simulink library "WrightSolverLib"  (R2014b)
settings: Solver=ode45  SolverMode=SingleTasking  StartTime=0.0  StopTime=10.0  RelTol=1e-3
undefined symbols (not defined in the file): BooleanThreshold, FloatingVoltage, FspSamplingPeriod, InfiniteResistance, NoCurrentOverride, WrightSolverSamplingPeriod
libraries: WrightSolverLib x34, simulink x5
settings Model: Creator=SWright2  LastModifiedBy=sj3-wright

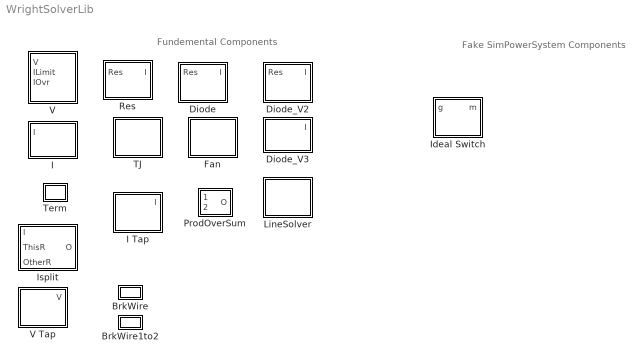
== system WrightSolverLib ==
  note: Fundemental Components
  note: Fake SimPowerSystem Components
  BrkWire : Subsystem
  BrkWire1to2 : Subsystem
  Diode : Subsystem
  Diode_V2 : Subsystem
  Diode_V3 : Subsystem
  Fan : Subsystem  RTWFcnName=TJunction  RTWFileName=TJunction
      settings: RTWFcnNameOpts=User specified  RTWFileNameOpts=User specified
  I : Subsystem
  I Tap : Subsystem
  Ideal Switch : Subsystem  mask{OnResistance=1}
  Isplit : Subsystem  RTWFcnName=Isplit  RTWFileName=Isplit
      settings: RTWFcnNameOpts=User specified  RTWFileNameOpts=User specified
  LineSolver : Subsystem
  ProdOverSum : Subsystem  RTWFcnName=ProdOverSum  RTWFileName=ProdOverSum
      settings: RTWFcnNameOpts=User specified  RTWFileNameOpts=User specified
  Res : Subsystem
  TJ : Subsystem  RTWFcnName=TJunction  RTWFileName=TJunction
      settings: RTWFcnNameOpts=User specified  RTWFileNameOpts=User specified
  Term : Subsystem
  V : Subsystem
  V Tap : Subsystem

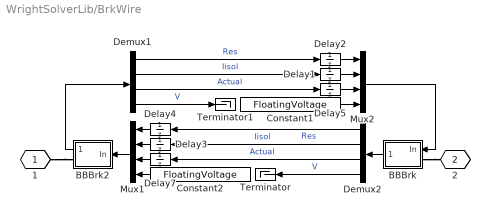
== system WrightSolverLib/BrkWire ==
  BBBrk : Subsystem
  BBBrk2 : Subsystem
  Constant1 : Constant  Value=FloatingVoltage
  Constant2 : Constant  Value=FloatingVoltage
  Delay{1,3,5,7} (4 alike) : UnitDelay  SampleTime=WrightSolverSamplingPeriod
  Delay2 : UnitDelay  InitialCondition=InfiniteResistance  SampleTime=WrightSolverSamplingPeriod
  Delay4 : UnitDelay  InitialCondition=InfiniteResistance  SampleTime=WrightSolverSamplingPeriod
  Demux1 : Demux
  Demux2 : Demux
  Mux1 : Mux
  Mux2 : Mux
  Terminator : Terminator
  Terminator1 : Terminator
  1 : PMIOPort  Tag=PMCPort  Port=1  Side=Left
  2 : PMIOPort  Tag=PMCPort  Port=2  Side=Right
  wires:
  BBBrk/1(Out) -> Demux2/1
  Demux2/3 -> Delay7/1  "Actual"
  Demux2/2 -> Delay3/1  "Iisol"
  Demux2/1 -> Delay4/1  "Res"
  Demux2/4 -> Terminator/1  "V"
  Mux1/1 -> BBBrk2/1(In)
  BBBrk2/1(Out) -> Demux1/1
  Mux2/1 -> BBBrk/1(In)
  Constant2/1 -> Mux1/4
  Delay4/1 -> Mux1/1
  Delay3/1 -> Mux1/2
  Delay7/1 -> Mux1/3
  Delay2/1 -> Mux2/1
  Delay1/1 -> Mux2/2
  Delay5/1 -> Mux2/3
  Constant1/1 -> Mux2/4
  Demux1/1 -> Delay2/1  "Res"
  Demux1/2 -> Delay1/1  "Iisol"
  Demux1/3 -> Delay5/1  "Actual"
  Demux1/4 -> Terminator1/1  "V"
  connections:
  BBBrk/LConn1 -- 2/RConn1
  1/RConn1 -- BBBrk2/RConn1

== system WrightSolverLib/BrkWire1to2 ==
  BBBrk : Subsystem
  BBBrk2 : Subsystem
  Delay : UnitDelay  InitialCondition=[InfiniteResistance 0 0 FloatingVoltage]  SampleTime=FspSamplingPeriod
  1 : PMIOPort  Tag=PMCPort  Port=1  Side=Left
  2 : PMIOPort  Tag=PMCPort  Port=2  Side=Right
  wires:
  BBBrk/1(Out) -> BBBrk2/1(In)
  BBBrk2/1(Out) -> Delay/1
  Delay/1 -> BBBrk/1(In)
  connections:
  1/RConn1 -- BBBrk2/RConn1
  BBBrk/LConn1 -- 2/RConn1

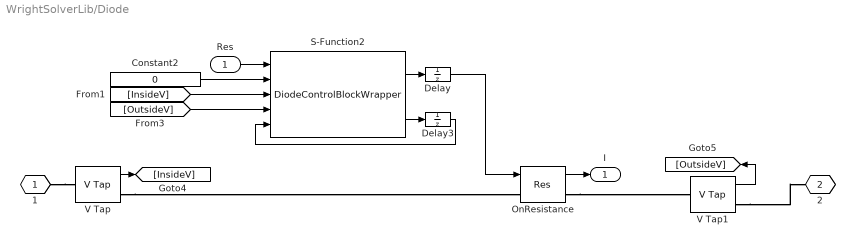
== system WrightSolverLib/Diode ==
  Res : Inport
  Constant2 : Constant  Value=0
  Delay : UnitDelay  InitialCondition=InfiniteResistance  SampleTime=-1
  Delay3 : UnitDelay  SampleTime=-1
  OnResistance : WrightSolverLib/Res
  S-Function2 : S-Function  FunctionName=DiodeControlBlockWrapper  EnableBusSupport=off
  V Tap : WrightSolverLib/V Tap
  V Tap1 : WrightSolverLib/V Tap
  1 : PMIOPort  Tag=PMCPort  Port=1  Side=Left
  2 : PMIOPort  Tag=PMCPort  Port=2  Side=Right
  I : Outport
  wires:
  V Tap1/1 -> [OutsideV]
  OnResistance/1 -> I/1
  V Tap/1 -> [InsideV]
  Constant2/1 -> S-Function2/2
  [InsideV] -> S-Function2/3
  S-Function2/1 -> Delay/1
  Res/1 -> S-Function2/1
  Delay/1 -> OnResistance/1
  S-Function2/2 -> Delay3/1
  Delay3/1 -> S-Function2/5
  [OutsideV] -> S-Function2/4
  connections:
  V Tap/RConn1 -- OnResistance/LConn1
  OnResistance/RConn1 -- V Tap1/LConn1
  1/RConn1 -- V Tap/LConn1
  V Tap1/RConn1 -- 2/RConn1

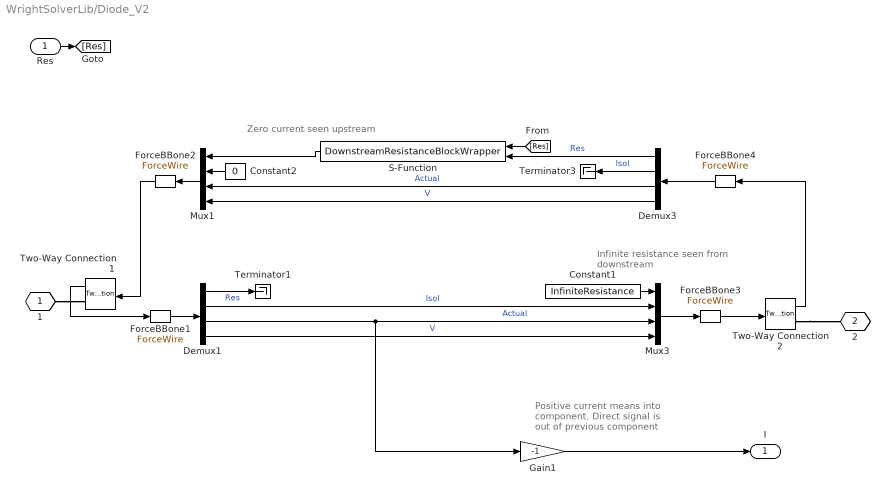
== system WrightSolverLib/Diode_V2 ==
  note: Positive current means
      | into component.
      | Direct signal is out
      | of previous
      | component
  note: Infinite
      | resistance
      | seen from
      | downstream
  note: Zero current
      | seen
      | upstream
  Res : Inport
  Constant1 : Constant  Value=InfiniteResistance
  Constant2 : Constant  Value=0
  Demux1 : Demux
  Demux3 : Demux
  ForceBBone{1..4} (4 alike) : WrightSolverLib/ForceWire
  Gain1 : Gain  Gain=-1
  Mux1 : Mux
  Mux3 : Mux
  S-Function : S-Function  FunctionName=DownstreamResistanceBlockWrapper  EnableBusSupport=off
  Terminator1 : Terminator
  Terminator3 : Terminator
  Two-Way Connection1 : TwoWayConnection
  Two-Way Connection2 : TwoWayConnection
  1 : PMIOPort  Tag=PMCPort  Port=1  Side=Left
  2 : PMIOPort  Tag=PMCPort  Port=2  Side=Right
  I : Outport
  wires:
  Gain1/1 -> I/1
  Demux3/3 -> Mux1/3  "Actual"
  Constant1/1 -> Mux3/1
  Res/1 -> [Res]
  Mux3/1 -> ForceBBone3/1
  Demux3/1 -> S-Function/2  "Res"
  Mux1/1 -> ForceBBone2/1
  S-Function/1 -> Mux1/1
  Two-Way Connection1/1 -> ForceBBone1/1
  Demux1/1 -> Terminator1/1  "Res"
  Demux3/2 -> Terminator3/1  "Isol"
  Demux1/2 -> Mux3/2  "Isol"
  Demux1/3 -> Gain1/1, Mux3/3  "Actual"
  ForceBBone2/1 -> Two-Way Connection1/1
  ForceBBone1/1 -> Demux1/1
  Constant2/1 -> Mux1/2
  Demux3/4 -> Mux1/4  "V"
  Demux1/4 -> Mux3/4  "V"
  Two-Way Connection2/1 -> ForceBBone4/1
  ForceBBone3/1 -> Two-Way Connection2/1
  ForceBBone4/1 -> Demux3/1
  [Res] -> S-Function/1
  connections:
  1/RConn1 -- Two-Way Connection1/RConn1
  Two-Way Connection2/RConn1 -- 2/RConn1

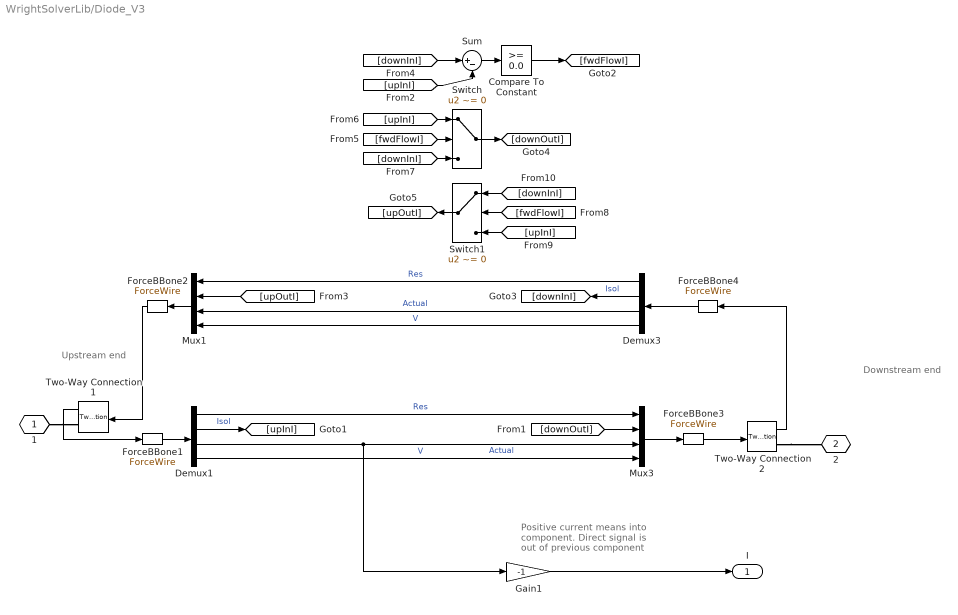
== system WrightSolverLib/Diode_V3 ==
  note: Positive current means
      | into component.
      | Direct signal is out
      | of previous
      | component
  note: Downstream
      | end
  note: Upstream
      | end
  Compare To Constant : simulink/Logic and Bit Operations/Compare To Constant  relop=>=  const=0.0  OutDataTypeStr=boolean
  Demux1 : Demux
  Demux3 : Demux
  ForceBBone{1..4} (4 alike) : WrightSolverLib/ForceWire
  Gain1 : Gain  Gain=-1
  Mux1 : Mux
  Mux3 : Mux
  Sum : Sum  Inputs=|+-
  Switch : Switch  Criteria=u2 ~= 0
  Switch1 : Switch  Criteria=u2 ~= 0
  Two-Way Connection1 : TwoWayConnection
  Two-Way Connection2 : TwoWayConnection
  1 : PMIOPort  Tag=PMCPort  Port=1  Side=Left
  2 : PMIOPort  Tag=PMCPort  Port=2  Side=Right
  I : Outport
  wires:
  Compare To Constant/1 -> [fwdFlowI]
  Sum/1 -> Compare To Constant/1
  [upInI] -> Sum/2
  [downInI] -> Sum/1
  ForceBBone4/1 -> Demux3/1
  ForceBBone3/1 -> Two-Way Connection2/1
  Two-Way Connection2/1 -> ForceBBone4/1
  Demux1/4 -> Mux3/4  "V"
  Demux3/4 -> Mux1/4  "V"
  [upOutI] -> Mux1/2
  ForceBBone1/1 -> Demux1/1
  ForceBBone2/1 -> Two-Way Connection1/1
  Demux1/3 -> Mux3/3, Gain1/1  "Actual"
  Demux3/2 -> [downInI]  "Isol"
  Demux1/1 -> Mux3/1  "Res"
  Two-Way Connection1/1 -> ForceBBone1/1
  Mux1/1 -> ForceBBone2/1
  Demux3/1 -> Mux1/1  "Res"
  Mux3/1 -> ForceBBone3/1
  Demux3/3 -> Mux1/3  "Actual"
  Gain1/1 -> I/1
  Demux1/2 -> [upInI]  "Isol"
  [downOutI] -> Mux3/2
  [fwdFlowI] -> Switch/2
  Switch/1 -> [downOutI]
  [upInI] -> Switch/1
  [downInI] -> Switch/3
  [fwdFlowI] -> Switch1/2
  Switch1/1 -> [upOutI]
  [downInI] -> Switch1/1
  [upInI] -> Switch1/3
  connections:
  Two-Way Connection2/RConn1 -- 2/RConn1
  1/RConn1 -- Two-Way Connection1/RConn1

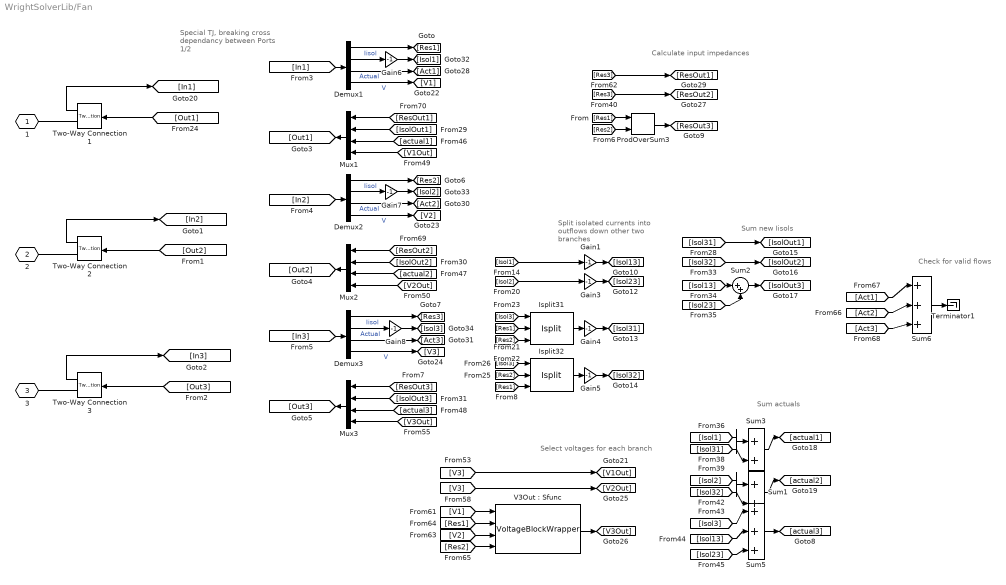
== system WrightSolverLib/Fan ==
  note: Check for valid flows
  note: Select voltages for each branch
  note: Calculate input impedances
  note: Split isolated currents
      | into outflows down other two
      | branches
  note: Sum new Iisols
  note: Sum actuals
  note: Special TJ, breaking
      | cross dependancy
      | between Ports 1/2
  Demux1 : Demux
  Demux2 : Demux
  Demux3 : Demux
  Gain{1,3..8} (7 alike) : Gain  Gain=-1
  Isplit31 : WrightSolverLib/Isplit
  Isplit32 : WrightSolverLib/Isplit
  Mux1 : Mux
  Mux2 : Mux
  Mux3 : Mux
  ProdOverSum3 : WrightSolverLib/ProdOverSum
  Sum1 : Sum  Inputs=|++
  Sum2 : Sum  Inputs=|++
  Sum3 : Sum  Inputs=|++
  Sum5 : Sum  Inputs=|+++
  Sum6 : Sum  Inputs=|+++
  Terminator1 : Terminator
  Two-Way Connection1 : TwoWayConnection
  Two-Way Connection2 : TwoWayConnection
  Two-Way Connection3 : TwoWayConnection
  "V3Out : Sfunc" : S-Function  FunctionName=VoltageBlockWrapper  EnableBusSupport=off
  1 : PMIOPort  Tag=PMCPort  Port=1  Side=Left
  2 : PMIOPort  Tag=PMCPort  Port=2  Side=Left
  3 : PMIOPort  Tag=PMCPort  Port=3  Side=Right
  wires:
  Sum6/1 -> Terminator1/1
  [Act3] -> Sum6/3
  [Act2] -> Sum6/2
  [Act1] -> Sum6/1
  Sum5/1 -> [actual3]
  Sum1/1 -> [actual2]
  Sum3/1 -> [actual1]
  "V3Out : Sfunc"/1 -> [V3Out]
  [Res2] -> "V3Out : Sfunc"/4
  [Res1] -> "V3Out : Sfunc"/2
  [V2] -> "V3Out : Sfunc"/3
  [V1] -> "V3Out : Sfunc"/1
  [V3] -> [V2Out]
  [V3] -> [V1Out]
  [V3Out] -> Mux3/4
  [V2Out] -> Mux2/4
  [V1Out] -> Mux1/4
  Mux1/1 -> [Out1]
  Mux2/1 -> [Out2]
  Mux3/1 -> [Out3]
  Demux1/1 -> [Res1]
  [Res1] -> ProdOverSum3/1
  Demux2/1 -> [Res2]
  Demux3/1 -> [Res3]
  [Res2] -> ProdOverSum3/2
  [ResOut3] -> Mux3/1
  ProdOverSum3/1 -> [ResOut3]
  [Res3] -> [ResOut2]
  [Res3] -> [ResOut1]
  [ResOut2] -> Mux2/1
  [ResOut1] -> Mux1/1
  Demux1/2 -> Gain6/1  "Iisol"
  Demux2/2 -> Gain7/1  "Iisol"
  Demux3/2 -> Gain8/1  "Iisol"
  [Isol1] -> Gain1/1
  [Isol3] -> Isplit31/1
  [Res1] -> Isplit31/2
  [Res2] -> Isplit31/3
  [Isol3] -> Isplit32/1
  [Res2] -> Isplit32/2
  [Res1] -> Isplit32/3
  [Isol31] -> [IsolOut1]
  [IsolOut1] -> Mux1/2
  [IsolOut2] -> Mux2/2
  [IsolOut3] -> Mux3/2
  [Isol32] -> [IsolOut2]
  [Isol13] -> Sum2/1
  Sum2/1 -> [IsolOut3]
  [Isol23] -> Sum2/2
  [Isol1] -> Sum3/1
  [Isol31] -> Sum3/2
  [Isol2] -> Sum1/1
  [Isol32] -> Sum1/2
  [Isol3] -> Sum5/1
  [Isol13] -> Sum5/2
  [Isol23] -> Sum5/3
  [actual1] -> Mux1/3
  [actual2] -> Mux2/3
  [actual3] -> Mux3/3
  Gain1/1 -> [Isol13]
  Gain3/1 -> [Isol23]
  Isplit31/1 -> Gain4/1
  Gain4/1 -> [Isol31]
  Isplit32/1 -> Gain5/1
  Gain5/1 -> [Isol32]
  Demux1/3 -> [Act1]  "Actual"
  Demux1/4 -> [V1]  "V"
  Demux2/3 -> [Act2]  "Actual"
  Demux2/4 -> [V2]  "V"
  Demux3/3 -> [Act3]  "Actual"
  Demux3/4 -> [V3]  "V"
  Gain6/1 -> [Isol1]
  Gain7/1 -> [Isol2]
  Gain8/1 -> [Isol3]
  [In1] -> Demux1/1
  [In2] -> Demux2/1
  [In3] -> Demux3/1
  [Out1] -> Two-Way Connection1/1
  [Out2] -> Two-Way Connection2/1
  [Out3] -> Two-Way Connection3/1
  Two-Way Connection1/1 -> [In1]
  Two-Way Connection2/1 -> [In2]
  Two-Way Connection3/1 -> [In3]
  [Isol2] -> Gain3/1
  connections:
  1/RConn1 -- Two-Way Connection1/RConn1
  2/RConn1 -- Two-Way Connection2/RConn1
  3/RConn1 -- Two-Way Connection3/RConn1

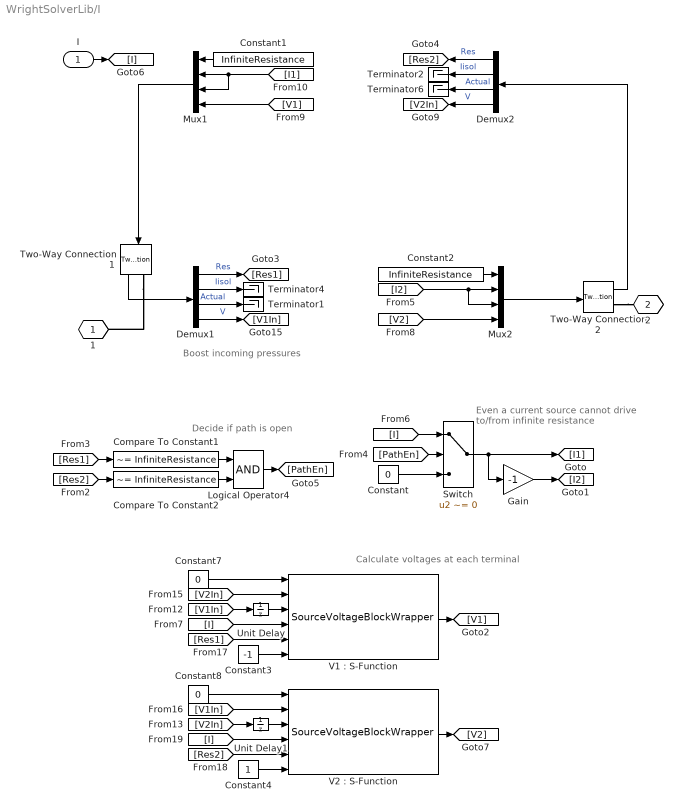
== system WrightSolverLib/I ==
  note: Calculate voltages at each terminal
  note: Decide if path is open
  note: Boost incoming
      | pressures
  note: Even a current source cannot drive
      | to/from infinite resistance
  I : Inport
  Compare To Constant1 : simulink/Logic and Bit Operations/Compare To Constant  relop=~=  const=InfiniteResistance  OutDataTypeStr=uint8  ZeroCross=off
  Compare To Constant2 : simulink/Logic and Bit Operations/Compare To Constant  relop=~=  const=InfiniteResistance  OutDataTypeStr=uint8  ZeroCross=off
  Constant : Constant  Value=0  OutDataTypeStr=Inherit: Inherit via back propagation
  Constant1 : Constant  Value=InfiniteResistance
  Constant2 : Constant  Value=InfiniteResistance
  Constant3 : Constant  Value=-1  OutDataTypeStr=Inherit: Inherit via back propagation
  Constant4 : Constant  OutDataTypeStr=Inherit: Inherit via back propagation
  Constant7 : Constant  Value=0  OutDataTypeStr=Inherit: Inherit via back propagation
  Constant8 : Constant  Value=0  OutDataTypeStr=Inherit: Inherit via back propagation
  Demux1 : Demux
  Demux2 : Demux
  Gain : Gain  Gain=-1
  Logical Operator4 : Logic  AllPortsSameDT=off  OutDataTypeStr=boolean
  Mux1 : Mux
  Mux2 : Mux
  Switch : Switch  Criteria=u2 ~= 0
  Terminator{1..2,4,6} (4 alike) : Terminator
  Two-Way Connection1 : TwoWayConnection
  Two-Way Connection2 : TwoWayConnection
  Unit Delay : UnitDelay  SampleTime=-1
  Unit Delay1 : UnitDelay  SampleTime=-1
  "V1 : S-Function" : S-Function  FunctionName=SourceVoltageBlockWrapper  EnableBusSupport=off
  "V2 : S-Function" : S-Function  FunctionName=SourceVoltageBlockWrapper  EnableBusSupport=off
  1 : PMIOPort  Tag=PMCPort  Port=1  Side=Left
  2 : PMIOPort  Tag=PMCPort  Port=2  Side=Right
  wires:
  [V2In] -> Unit Delay1/1
  "V2 : S-Function"/1 -> [V2]
  [V1In] -> Unit Delay/1
  Logical Operator4/1 -> [PathEn]
  Mux2/1 -> Two-Way Connection2/1
  Two-Way Connection2/1 -> Demux2/1
  Demux1/3 -> Terminator1/1  "Actual"
  Demux2/3 -> Terminator6/1  "Actual"
  Demux2/2 -> Terminator2/1  "Iisol"
  [I2] -> Mux2/2, Mux2/3
  Constant1/1 -> Mux1/1
  Demux2/1 -> [Res2]  "Res"
  Demux1/2 -> Terminator4/1  "Iisol"
  Constant2/1 -> Mux2/1
  Demux1/1 -> [Res1]  "Res"
  Mux1/1 -> Two-Way Connection1/1
  Two-Way Connection1/1 -> Demux1/1
  Demux2/4 -> [V2In]  "V"
  Demux1/4 -> [V1In]  "V"
  Compare To Constant1/1 -> Logical Operator4/1
  Compare To Constant2/1 -> Logical Operator4/2
  [Res1] -> Compare To Constant1/1
  [Res2] -> Compare To Constant2/1
  [PathEn] -> Switch/2
  Switch/1 -> [I1], Gain/1
  [I] -> Switch/1
  Constant/1 -> Switch/3
  [V1] -> Mux1/4
  [I1] -> Mux1/2, Mux1/3
  [V2] -> Mux2/4
  Gain/1 -> [I2]
  I/1 -> [I]
  [Res1] -> "V1 : S-Function"/5
  [I] -> "V1 : S-Function"/4
  "V1 : S-Function"/1 -> [V1]
  [Res2] -> "V2 : S-Function"/5
  [I] -> "V2 : S-Function"/4
  Constant3/1 -> "V1 : S-Function"/6
  Constant4/1 -> "V2 : S-Function"/6
  Constant7/1 -> "V1 : S-Function"/1
  Constant8/1 -> "V2 : S-Function"/1
  [V2In] -> "V1 : S-Function"/2
  [V1In] -> "V2 : S-Function"/2
  Unit Delay/1 -> "V1 : S-Function"/3
  Unit Delay1/1 -> "V2 : S-Function"/3
  connections:
  Two-Way Connection1/RConn1 -- 1/RConn1
  Two-Way Connection2/RConn1 -- 2/RConn1

== system WrightSolverLib/I Tap ==
  note: Positive current means
      | into component.
      | Direct signal is out
      | of previous
      | component
  Demux1 : Demux
  Gain7 : Gain  Gain=-1
  Mux3 : Mux
  Two-Way Connection1 : TwoWayConnection
  Two-Way Connection2 : TwoWayConnection
  1 : PMIOPort  Tag=PMCPort  Port=1  Side=Left
  2 : PMIOPort  Tag=PMCPort  Port=2  Side=Right
  I : Outport
  wires:
  Mux3/1 -> Two-Way Connection2/1
  Two-Way Connection2/1 -> Two-Way Connection1/1
  Demux1/1 -> Mux3/1
  Demux1/2 -> Mux3/2  "Iisol"
  Demux1/3 -> Mux3/3, Gain7/1
  Two-Way Connection1/1 -> Demux1/1
  Demux1/4 -> Mux3/4
  Gain7/1 -> I/1
  connections:
  1/RConn1 -- Two-Way Connection1/RConn1
  Two-Way Connection2/RConn1 -- 2/RConn1

== system WrightSolverLib/Ideal Switch ==
  g : Inport
  Constant1 : Constant  Value=OnResistance
  Constant6 : Constant  Value=InfiniteResistance
  Res : WrightSolverLib/Res
  Switch1 : Switch  Threshold=BooleanThreshold
  1 : PMIOPort  Tag=PMCPort  Port=1  Side=Left
  2 : PMIOPort  Tag=PMCPort  Port=2  Side=Right
  m : Outport
  wires:
  Res/1 -> m/1
  Switch1/1 -> Res/1
  Constant6/1 -> Switch1/3
  g/1 -> Switch1/2
  Constant1/1 -> Switch1/1
  connections:
  1/RConn1 -- Res/LConn1
  Res/RConn1 -- 2/RConn1

== system WrightSolverLib/Isplit ==
  note: Splits current by R2/(R1+R2)
  I : Inport
  ThisR : Inport  Port=2
  OtherR : Inport  Port=3
  S-Function : S-Function  FunctionName=CurrentSplitBlockWrapper  EnableBusSupport=off
  O : Outport
  wires:
  I/1 -> S-Function/1
  OtherR/1 -> S-Function/3
  ThisR/1 -> S-Function/2
  S-Function/1 -> O/1

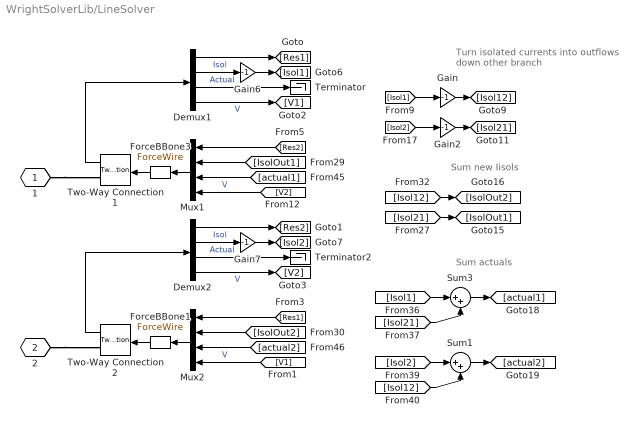
== system WrightSolverLib/LineSolver ==
  note: Turn isolated currents
      | into outflows down other branch
  note: Sum new Iisols
  note: Sum actuals
  Demux1 : Demux
  Demux2 : Demux
  ForceBBone1 : WrightSolverLib/ForceWire
  ForceBBone3 : WrightSolverLib/ForceWire
  Gain{,2,6..7} (4 alike) : Gain  Gain=-1
  Mux1 : Mux
  Mux2 : Mux
  Sum1 : Sum  Inputs=|++
  Sum3 : Sum  Inputs=|++
  Terminator : Terminator
  Terminator2 : Terminator
  Two-Way Connection1 : TwoWayConnection
  Two-Way Connection2 : TwoWayConnection
  1 : PMIOPort  Tag=PMCPort  Port=1  Side=Left
  2 : PMIOPort  Tag=PMCPort  Port=2  Side=Right
  wires:
  Two-Way Connection1/1 -> Demux1/1
  Mux1/1 -> ForceBBone3/1
  Two-Way Connection2/1 -> Demux2/1
  Mux2/1 -> ForceBBone1/1
  Demux1/1 -> [Res1]
  Demux2/1 -> [Res2]
  [Res1] -> Mux2/1
  [Res2] -> Mux1/1
  Demux1/2 -> Gain6/1  "Isol"
  Demux2/2 -> Gain7/1  "Isol"
  [Isol1] -> Gain/1
  [Isol2] -> Gain2/1
  [Isol21] -> [IsolOut1]
  [IsolOut1] -> Mux1/2
  [IsolOut2] -> Mux2/2
  [Isol12] -> [IsolOut2]
  [Isol1] -> Sum3/1
  Sum3/1 -> [actual1]
  [Isol21] -> Sum3/2
  [Isol2] -> Sum1/1
  Sum1/1 -> [actual2]
  [Isol12] -> Sum1/2
  [actual1] -> Mux1/3
  [actual2] -> Mux2/3
  Gain/1 -> [Isol12]
  Gain2/1 -> [Isol21]
  Demux1/3 -> Terminator/1  "Actual"
  Demux1/4 -> [V1]  "V"
  Demux2/3 -> Terminator2/1  "Actual"
  Demux2/4 -> [V2]  "V"
  [V1] -> Mux2/4  "V"
  Gain6/1 -> [Isol1]
  Gain7/1 -> [Isol2]
  ForceBBone3/1 -> Two-Way Connection1/1
  ForceBBone1/1 -> Two-Way Connection2/1
  [V2] -> Mux1/4  "V"
  connections:
  1/RConn1 -- Two-Way Connection1/RConn1
  2/RConn1 -- Two-Way Connection2/RConn1

== system WrightSolverLib/ProdOverSum ==
  note: Product-over-sum, including
      | infinity interception. Used for
      | calculating parallel resistances
  1 : Inport
  2 : Inport  Port=2
  S-Function : S-Function  FunctionName=ParallelResistanceBlockWrapper  EnableBusSupport=off
  O : Outport
  wires:
  1/1 -> S-Function/1
  2/1 -> S-Function/2
  S-Function/1 -> O/1

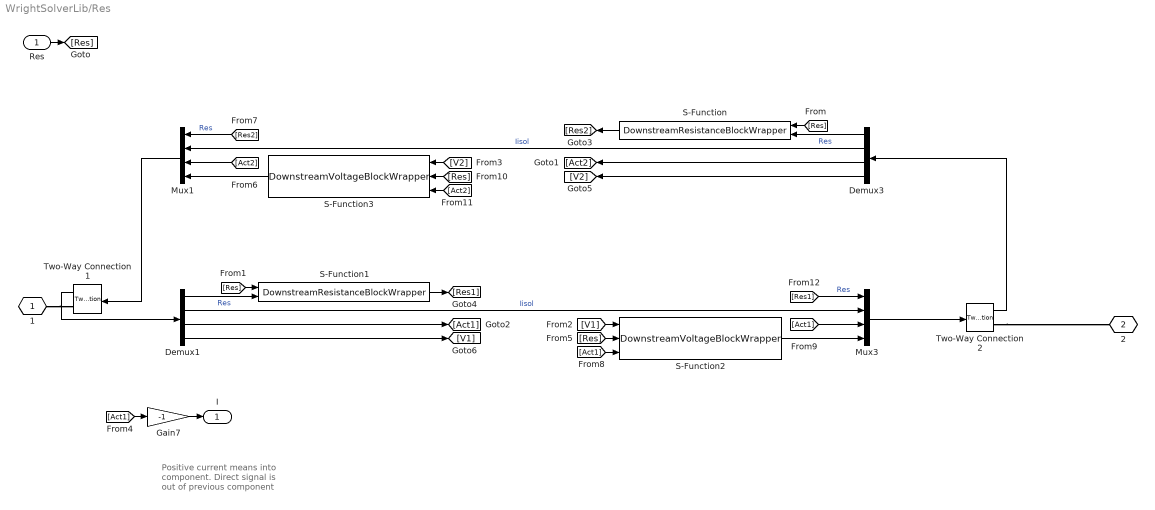
== system WrightSolverLib/Res ==
  note: Positive current means
      | into component.
      | Direct signal is out
      | of previous
      | component
  Res : Inport
  Demux1 : Demux
  Demux3 : Demux
  Gain7 : Gain  Gain=-1
  Mux1 : Mux
  Mux3 : Mux
  S-Function : S-Function  FunctionName=DownstreamResistanceBlockWrapper  EnableBusSupport=off
  S-Function1 : S-Function  FunctionName=DownstreamResistanceBlockWrapper  EnableBusSupport=off
  S-Function2 : S-Function  FunctionName=DownstreamVoltageBlockWrapper  EnableBusSupport=off
  S-Function3 : S-Function  FunctionName=DownstreamVoltageBlockWrapper  EnableBusSupport=off
  Two-Way Connection1 : TwoWayConnection
  Two-Way Connection2 : TwoWayConnection
  1 : PMIOPort  Tag=PMCPort  Port=1  Side=Left
  2 : PMIOPort  Tag=PMCPort  Port=2  Side=Right
  I : Outport
  wires:
  Res/1 -> [Res]
  Demux3/1 -> S-Function/2  "Res"
  [Res] -> S-Function1/1
  Demux1/1 -> S-Function1/2  "Res"
  Demux3/3 -> [Act2]
  Demux1/3 -> [Act1]
  Mux1/1 -> Two-Way Connection1/1
  Two-Way Connection1/1 -> Demux1/1
  Mux3/1 -> Two-Way Connection2/1
  Two-Way Connection2/1 -> Demux3/1
  [Res] -> S-Function/1
  Gain7/1 -> I/1
  [Act1] -> Gain7/1
  [Act2] -> Mux1/3
  S-Function/1 -> [Res2]
  [Res2] -> Mux1/1  "Res"
  S-Function1/1 -> [Res1]
  [Res1] -> Mux3/1  "Res"
  [Act1] -> Mux3/3
  Demux3/4 -> [V2]
  S-Function2/1 -> Mux3/4
  Demux1/4 -> [V1]
  [V1] -> S-Function2/1
  [Res] -> S-Function2/2
  [Act1] -> S-Function2/3
  [V2] -> S-Function3/1
  [Res] -> S-Function3/2
  [Act2] -> S-Function3/3
  S-Function3/1 -> Mux1/4
  Demux1/2 -> Mux3/2  "Iisol"
  Demux3/2 -> Mux1/2  "Iisol"
  connections:
  1/RConn1 -- Two-Way Connection1/RConn1
  Two-Way Connection2/RConn1 -- 2/RConn1

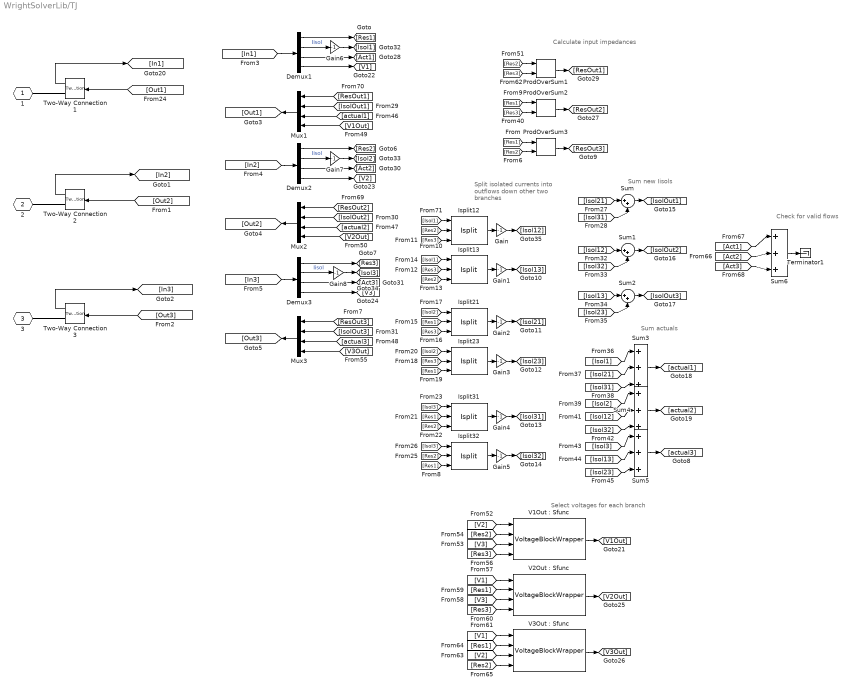
== system WrightSolverLib/TJ ==
  note: Sum actuals
  note: Sum new Iisols
  note: Split isolated currents
      | into outflows down other two
      | branches
  note: Calculate input impedances
  note: Select voltages for each branch
  note: Check for valid flows
  Demux1 : Demux
  Demux2 : Demux
  Demux3 : Demux
  Gain{,1..8} (9 alike) : Gain  Gain=-1
  Isplit{12..13,21,23,31..32} (6 alike) : WrightSolverLib/Isplit
  Mux1 : Mux
  Mux2 : Mux
  Mux3 : Mux
  ProdOverSum1 : WrightSolverLib/ProdOverSum
  ProdOverSum2 : WrightSolverLib/ProdOverSum
  ProdOverSum3 : WrightSolverLib/ProdOverSum
  Sum : Sum  Inputs=|++
  Sum1 : Sum  Inputs=|++
  Sum2 : Sum  Inputs=|++
  Sum{3..6} (4 alike) : Sum  Inputs=|+++
  Terminator1 : Terminator
  Two-Way Connection1 : TwoWayConnection
  Two-Way Connection2 : TwoWayConnection
  Two-Way Connection3 : TwoWayConnection
  "V1Out : Sfunc" : S-Function  FunctionName=VoltageBlockWrapper  EnableBusSupport=off
  "V2Out : Sfunc" : S-Function  FunctionName=VoltageBlockWrapper  EnableBusSupport=off
  "V3Out : Sfunc" : S-Function  FunctionName=VoltageBlockWrapper  EnableBusSupport=off
  1 : PMIOPort  Tag=PMCPort  Port=1  Side=Left
  2 : PMIOPort  Tag=PMCPort  Port=2  Side=Right
  3 : PMIOPort  Tag=PMCPort  Port=3  Side=Right
  wires:
  [In3] -> Demux3/1
  [In2] -> Demux2/1
  [In1] -> Demux1/1
  Two-Way Connection3/1 -> [In3]
  Two-Way Connection2/1 -> [In2]
  Two-Way Connection1/1 -> [In1]
  [Out3] -> Two-Way Connection3/1
  [Out2] -> Two-Way Connection2/1
  [Out1] -> Two-Way Connection1/1
  Gain8/1 -> [Isol3]
  Gain7/1 -> [Isol2]
  Gain6/1 -> [Isol1]
  Demux3/4 -> [V3]
  Demux3/3 -> [Act3]
  Demux2/4 -> [V2]
  Demux2/3 -> [Act2]
  Demux1/4 -> [V1]
  Demux1/3 -> [Act1]
  Gain5/1 -> [Isol32]
  Isplit32/1 -> Gain5/1
  Gain4/1 -> [Isol31]
  Isplit31/1 -> Gain4/1
  Isplit23/1 -> Gain3/1
  Gain3/1 -> [Isol23]
  Gain2/1 -> [Isol21]
  Isplit21/1 -> Gain2/1
  Isplit13/1 -> Gain1/1
  Gain1/1 -> [Isol13]
  Gain/1 -> [Isol12]
  [actual3] -> Mux3/3
  [actual2] -> Mux2/3
  [actual1] -> Mux1/3
  [Isol23] -> Sum5/3
  [Isol13] -> Sum5/2
  [Isol3] -> Sum5/1
  [Isol32] -> Sum4/3
  [Isol12] -> Sum4/2
  [Isol2] -> Sum4/1
  [Isol31] -> Sum3/3
  [Isol21] -> Sum3/2
  [Isol1] -> Sum3/1
  [Isol23] -> Sum2/2
  Sum2/1 -> [IsolOut3]
  [Isol13] -> Sum2/1
  [Isol32] -> Sum1/2
  Sum1/1 -> [IsolOut2]
  [Isol12] -> Sum1/1
  [IsolOut3] -> Mux3/2
  [IsolOut2] -> Mux2/2
  [IsolOut1] -> Mux1/2
  [Isol31] -> Sum/2
  Sum/1 -> [IsolOut1]
  [Isol21] -> Sum/1
  [Res1] -> Isplit32/3
  [Res2] -> Isplit32/2
  [Isol3] -> Isplit32/1
  [Res2] -> Isplit31/3
  [Res1] -> Isplit31/2
  [Isol3] -> Isplit31/1
  [Res1] -> Isplit23/3
  [Res3] -> Isplit23/2
  [Isol2] -> Isplit23/1
  [Res3] -> Isplit21/3
  [Res1] -> Isplit21/2
  [Isol2] -> Isplit21/1
  [Res2] -> Isplit13/3
  [Res3] -> Isplit13/2
  [Isol1] -> Isplit13/1
  Isplit12/1 -> Gain/1
  [Res3] -> Isplit12/3
  [Res2] -> Isplit12/2
  [Isol1] -> Isplit12/1
  Demux3/2 -> Gain8/1  "Iisol"
  Demux2/2 -> Gain7/1  "Iisol"
  Demux1/2 -> Gain6/1  "Iisol"
  [ResOut1] -> Mux1/1
  [ResOut2] -> Mux2/1
  ProdOverSum1/1 -> [ResOut1]
  [Res3] -> ProdOverSum1/2
  [Res2] -> ProdOverSum1/1
  ProdOverSum2/1 -> [ResOut2]
  [Res3] -> ProdOverSum2/2
  [Res1] -> ProdOverSum2/1
  ProdOverSum3/1 -> [ResOut3]
  [ResOut3] -> Mux3/1
  [Res2] -> ProdOverSum3/2
  Demux3/1 -> [Res3]
  Demux2/1 -> [Res2]
  [Res1] -> ProdOverSum3/1
  Demux1/1 -> [Res1]
  Mux3/1 -> [Out3]
  Mux2/1 -> [Out2]
  Mux1/1 -> [Out1]
  [V1Out] -> Mux1/4
  [V2Out] -> Mux2/4
  [V3Out] -> Mux3/4
  [V2] -> "V1Out : Sfunc"/1
  [V3] -> "V1Out : Sfunc"/3
  [Res2] -> "V1Out : Sfunc"/2
  [Res3] -> "V1Out : Sfunc"/4
  "V1Out : Sfunc"/1 -> [V1Out]
  [V1] -> "V2Out : Sfunc"/1
  [V3] -> "V2Out : Sfunc"/3
  [Res1] -> "V2Out : Sfunc"/2
  [Res3] -> "V2Out : Sfunc"/4
  "V2Out : Sfunc"/1 -> [V2Out]
  [V1] -> "V3Out : Sfunc"/1
  [V2] -> "V3Out : Sfunc"/3
  [Res1] -> "V3Out : Sfunc"/2
  [Res2] -> "V3Out : Sfunc"/4
  "V3Out : Sfunc"/1 -> [V3Out]
  Sum3/1 -> [actual1]
  Sum4/1 -> [actual2]
  Sum5/1 -> [actual3]
  [Act1] -> Sum6/1
  [Act2] -> Sum6/2
  [Act3] -> Sum6/3
  Sum6/1 -> Terminator1/1
  connections:
  3/RConn1 -- Two-Way Connection3/RConn1
  2/RConn1 -- Two-Way Connection2/RConn1
  1/RConn1 -- Two-Way Connection1/RConn1

== system WrightSolverLib/Term ==
  note: Retransmit
      | actual
      | flow
  Constant1 : Constant  Value=0
  Constant2 : Constant  Value=0
  Constant4 : Constant  Value=0
  Demux1 : Demux
  Gain7 : Gain  Gain=-1
  Mux1 : Mux
  Terminator : Terminator
  Terminator1 : Terminator
  Terminator2 : Terminator
  Two-Way Connection1 : TwoWayConnection
  1 : PMIOPort  Tag=PMCPort  Port=1  Side=Right
  wires:
  Two-Way Connection1/1 -> Demux1/1
  Constant4/1 -> Mux1/1
  Demux1/1 -> Terminator/1
  Constant1/1 -> Mux1/2  "Iisol"
  Demux1/2 -> Terminator1/1  "Iisol"
  Mux1/1 -> Two-Way Connection1/1
  Demux1/4 -> Terminator2/1
  Constant2/1 -> Mux1/4
  Gain7/1 -> Mux1/3
  Demux1/3 -> Gain7/1
  connections:
  Two-Way Connection1/RConn1 -- 1/RConn1

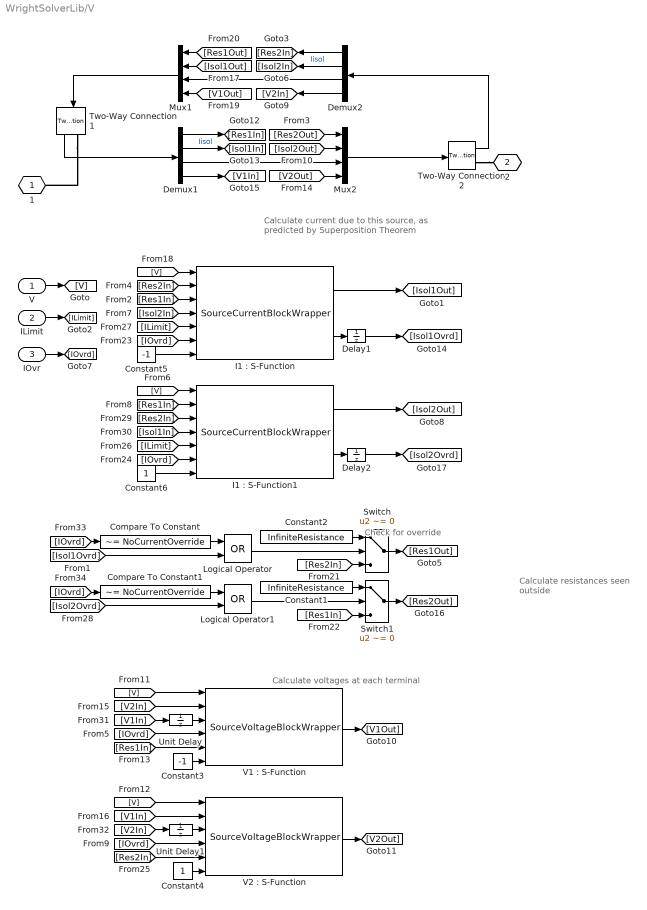
== system WrightSolverLib/V ==
  note: Calculate current due to this source,
      | as predicted by Superposition Theorem
  note: Calculate resistances
      | seen outside
  note: Check for override
  note: Calculate voltages at each terminal
  V : Inport
  ILimit : Inport  Port=2
  IOvr : Inport  Port=3
  Compare To Constant : simulink/Logic and Bit Operations/Compare To Constant  relop=~=  const=NoCurrentOverride  OutDataTypeStr=uint8  ZeroCross=off
  Compare To Constant1 : simulink/Logic and Bit Operations/Compare To Constant  relop=~=  const=NoCurrentOverride  OutDataTypeStr=uint8  ZeroCross=off
  Constant1 : Constant  Value=InfiniteResistance
  Constant2 : Constant  Value=InfiniteResistance
  Constant3 : Constant  Value=-1  OutDataTypeStr=Inherit: Inherit via back propagation
  Constant4 : Constant  OutDataTypeStr=Inherit: Inherit via back propagation
  Constant5 : Constant  Value=-1  OutDataTypeStr=Inherit: Inherit via back propagation
  Constant6 : Constant  OutDataTypeStr=Inherit: Inherit via back propagation
  Delay1 : UnitDelay  SampleTime=-1
  Delay2 : UnitDelay  SampleTime=-1
  Demux1 : Demux
  Demux2 : Demux
  "I1 : S-Function" : S-Function  FunctionName=SourceCurrentBlockWrapper  EnableBusSupport=off
  "I1 : S-Function1" : S-Function  FunctionName=SourceCurrentBlockWrapper  EnableBusSupport=off
  Logical Operator : Logic  Operator=OR  AllPortsSameDT=off  OutDataTypeStr=boolean
  Logical Operator1 : Logic  Operator=OR  AllPortsSameDT=off  OutDataTypeStr=boolean
  Mux1 : Mux
  Mux2 : Mux
  Switch : Switch  Criteria=u2 ~= 0
  Switch1 : Switch  Criteria=u2 ~= 0
  Two-Way Connection1 : TwoWayConnection
  Two-Way Connection2 : TwoWayConnection
  Unit Delay : UnitDelay  SampleTime=-1
  Unit Delay1 : UnitDelay  SampleTime=-1
  "V1 : S-Function" : S-Function  FunctionName=SourceVoltageBlockWrapper  EnableBusSupport=off
  "V2 : S-Function" : S-Function  FunctionName=SourceVoltageBlockWrapper  EnableBusSupport=off
  1 : PMIOPort  Tag=PMCPort  Port=1  Side=Left
  2 : PMIOPort  Tag=PMCPort  Port=2  Side=Right
  wires:
  Logical Operator1/1 -> Switch1/2
  [IOvrd] -> Compare To Constant1/1
  Compare To Constant1/1 -> Logical Operator1/1
  [Isol2Ovrd] -> Logical Operator1/2
  Logical Operator/1 -> Switch/2
  Compare To Constant/1 -> Logical Operator/1
  [Isol1Ovrd] -> Logical Operator/2
  Constant1/1 -> Switch1/1
  [IOvrd] -> Compare To Constant/1
  "I1 : S-Function1"/1 -> [Isol2Out]
  "I1 : S-Function1"/2 -> Delay2/1
  Delay2/1 -> [Isol2Ovrd]
  "I1 : S-Function"/1 -> [Isol1Out]
  Demux1/1 -> [Res1In]
  V/1 -> [V]
  [Res2Out] -> Mux2/1
  Demux1/2 -> [Isol1In]  "Iisol"
  Demux2/1 -> [Res2In]
  [Res1Out] -> Mux1/1
  [Isol2Out] -> Mux2/2
  [Isol1Out] -> Mux1/2
  Demux2/2 -> [Isol2In]  "Iisol"
  Mux2/1 -> Two-Way Connection2/1
  Two-Way Connection2/1 -> Demux2/1
  Two-Way Connection1/1 -> Demux1/1
  Mux1/1 -> Two-Way Connection1/1
  [V1Out] -> Mux1/4
  IOvr/1 -> [IOvrd]
  Demux2/4 -> [V2In]
  Demux2/3 -> Mux1/3
  Demux1/3 -> Mux2/3
  Demux1/4 -> [V1In]
  [V2Out] -> Mux2/4
  Switch/1 -> [Res1Out]
  Constant2/1 -> Switch/1
  [Res2In] -> Switch/3
  Switch1/1 -> [Res2Out]
  [Res1In] -> Switch1/3
  "V1 : S-Function"/1 -> [V1Out]
  [Res2In] -> "V2 : S-Function"/5
  [IOvrd] -> "V2 : S-Function"/4
  [V2In] -> Unit Delay1/1
  [V] -> "V2 : S-Function"/1
  Constant4/1 -> "V2 : S-Function"/6
  ILimit/1 -> [ILimit]
  "I1 : S-Function"/2 -> Delay1/1
  Delay1/1 -> [Isol1Ovrd]
  [V] -> "I1 : S-Function"/1
  [Res2In] -> "I1 : S-Function"/2
  [Res1In] -> "I1 : S-Function"/3
  [Isol2In] -> "I1 : S-Function"/4
  [ILimit] -> "I1 : S-Function"/5
  [IOvrd] -> "I1 : S-Function"/6
  [V] -> "I1 : S-Function1"/1
  [Res1In] -> "I1 : S-Function1"/2
  [Res2In] -> "I1 : S-Function1"/3
  [Isol1In] -> "I1 : S-Function1"/4
  [ILimit] -> "I1 : S-Function1"/5
  [IOvrd] -> "I1 : S-Function1"/6
  Constant5/1 -> "I1 : S-Function"/7
  Constant6/1 -> "I1 : S-Function1"/7
  [V] -> "V1 : S-Function"/1
  [V2In] -> "V1 : S-Function"/2
  [IOvrd] -> "V1 : S-Function"/4
  [Res1In] -> "V1 : S-Function"/5
  Constant3/1 -> "V1 : S-Function"/6
  [V1In] -> "V2 : S-Function"/2
  "V2 : S-Function"/1 -> [V2Out]
  Unit Delay/1 -> "V1 : S-Function"/3
  [V1In] -> Unit Delay/1
  Unit Delay1/1 -> "V2 : S-Function"/3
  connections:
  Two-Way Connection2/RConn1 -- 2/RConn1
  Two-Way Connection1/RConn1 -- 1/RConn1

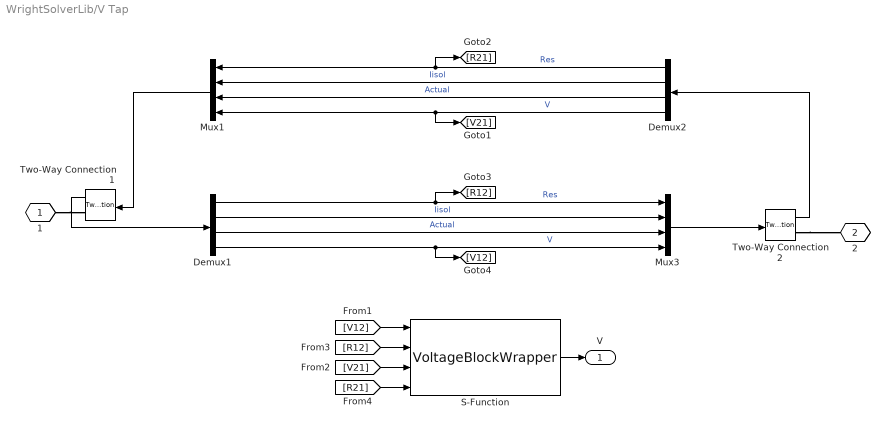
== system WrightSolverLib/V Tap ==
  Demux1 : Demux
  Demux2 : Demux
  Mux1 : Mux
  Mux3 : Mux
  S-Function : S-Function  FunctionName=VoltageBlockWrapper  EnableBusSupport=off
  Two-Way Connection1 : TwoWayConnection
  Two-Way Connection2 : TwoWayConnection
  1 : PMIOPort  Tag=PMCPort  Port=1  Side=Left
  2 : PMIOPort  Tag=PMCPort  Port=2  Side=Right
  V : Outport
  wires:
  Mux3/1 -> Two-Way Connection2/1
  Mux1/1 -> Two-Way Connection1/1
  Demux1/1 -> Mux3/1, [R12]  "Res"
  Demux1/2 -> Mux3/2  "Iisol"
  Demux1/3 -> Mux3/3  "Actual"
  Two-Way Connection1/1 -> Demux1/1
  Demux1/4 -> Mux3/4, [V12]  "V"
  Demux2/1 -> Mux1/1, [R21]  "Res"
  Demux2/2 -> Mux1/2  "Iisol"
  Demux2/3 -> Mux1/3  "Actual"
  Demux2/4 -> Mux1/4, [V21]  "V"
  Two-Way Connection2/1 -> Demux2/1
  [V12] -> S-Function/1
  S-Function/1 -> V/1
  [V21] -> S-Function/3
  [R12] -> S-Function/2
  [R21] -> S-Function/4
  connections:
  Two-Way Connection2/RConn1 -- 2/RConn1
  1/RConn1 -- Two-Way Connection1/RConn1

== system WrightSolverLib/BrkWire/BBBrk ==
  In : Inport
  ForceWireI : WrightSolverLib/ForceWire
  ForceWireO : WrightSolverLib/ForceWire
  Two-Way Connection1 : TwoWayConnection
  BB : PMIOPort  Tag=PMCPort  Port=1  Side=Left
  Out : Outport
  wires:
  ForceWireI/1 -> Two-Way Connection1/1
  ForceWireO/1 -> Out/1
  In/1 -> ForceWireI/1
  Two-Way Connection1/1 -> ForceWireO/1
  connections:
  BB/RConn1 -- Two-Way Connection1/RConn1

== system WrightSolverLib/BrkWire/BBBrk2 ==
  In : Inport
  ForceWireI : WrightSolverLib/ForceWire
  ForceWireO : WrightSolverLib/ForceWire
  Two-Way Connection1 : TwoWayConnection
  BB : PMIOPort  Tag=PMCPort  Port=1  Side=Right
  Out : Outport
  wires:
  ForceWireO/1 -> Out/1
  ForceWireI/1 -> Two-Way Connection1/1
  Two-Way Connection1/1 -> ForceWireO/1
  In/1 -> ForceWireI/1
  connections:
  BB/RConn1 -- Two-Way Connection1/RConn1

== system WrightSolverLib/BrkWire1to2/BBBrk ==
  In : Inport
  ForceWireI : WrightSolverLib/ForceWire
  ForceWireO : WrightSolverLib/ForceWire
  Two-Way Connection1 : TwoWayConnection
  BB : PMIOPort  Tag=PMCPort  Port=1  Side=Left
  Out : Outport
  wires:
  Two-Way Connection1/1 -> ForceWireO/1
  In/1 -> ForceWireI/1
  ForceWireO/1 -> Out/1
  ForceWireI/1 -> Two-Way Connection1/1
  connections:
  BB/RConn1 -- Two-Way Connection1/RConn1

== system WrightSolverLib/BrkWire1to2/BBBrk2 ==
  In : Inport
  ForceWireI : WrightSolverLib/ForceWire
  ForceWireO : WrightSolverLib/ForceWire
  Two-Way Connection1 : TwoWayConnection
  BB : PMIOPort  Tag=PMCPort  Port=1  Side=Right
  Out : Outport
  wires:
  In/1 -> ForceWireI/1
  Two-Way Connection1/1 -> ForceWireO/1
  ForceWireI/1 -> Two-Way Connection1/1
  ForceWireO/1 -> Out/1
  connections:
  BB/RConn1 -- Two-Way Connection1/RConn1
